simulink model "biox"  (Simulink 7.6)
settings: Solver=ode45  SolverMode=SingleTasking  StartTime=0.0  StopTime=200.0  MaxStep=0.1  RelTol=1e-9  AbsTol=1e-12
settings Model: Creator=fforbes  LastModifiedBy=fforbes  ExtModeTrigMode=oneshot  ExtModeArmWhenConnect=off
settings SolverCC: InitialStep=0.1
settings DataIOCC: LimitDataPoints=off
settings OptimizationCC: BlockReduction=off  BooleanDataType=off
settings DebuggingCC: SaveWithParameterizedLinksMsg=none  SignalResolutionControl=TryResolveAllWithWarning  SolverPrmCheckMsg=none  MultiTaskDSMMsg=warning  MultiTaskCondExecSysMsg=none  StrictBusMsg=None
settings HardwareCC: TargetUnknown=on
settings RTWCC: IncludeERTFirstTime=on

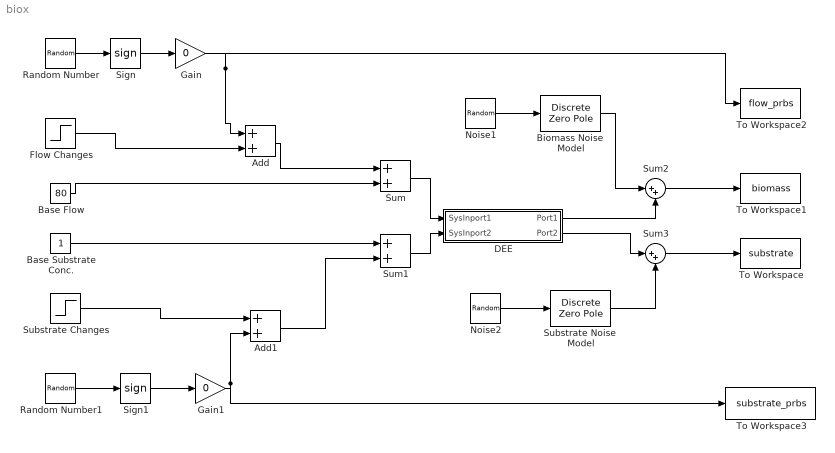
== system biox ==
  Add : Sum
  Add1 : Sum
  Base Flow : Constant  Value=80
  Base Substrate Conc. : Constant
  Biomass Noise  Model : DiscreteZeroPole  Zeros=[0.5]  Poles=[0 0.4 1]  Gain=.01
  DEE : Subsystem
      settings: OpenFcn=diffeqed
      mask Type: Differential Equation Editor (DEE)
      mask Display: disp('BIOX Unit')
  Flow Changes : Step  Time=5  After=0  SampleTime=0
  Gain : Gain  Gain=0
  Gain1 : Gain  Gain=0
  Noise1 : RandomNumber  Variance=0.00001  SampleTime=0.1
  Noise2 : RandomNumber  Variance=0.00000001  SampleTime=0.1
  Random Number : RandomNumber  SampleTime=1
  Random Number1 : RandomNumber  SampleTime=1
  Sign : Signum
  Sign1 : Signum
  Substrate Changes : Step  Time=5  After=0  SampleTime=0
  Substrate Noise  Model : DiscreteZeroPole  Zeros=[0.5]  Poles=[0.2 0.8]  Gain=1
  Sum : Sum  SaturateOnIntegerOverflow=on  InputSameDT=on  OutDataTypeStr=Inherit: Same as first input
  Sum1 : Sum  SaturateOnIntegerOverflow=on  InputSameDT=on  OutDataTypeStr=Inherit: Same as first input
  Sum2 : Sum  Inputs=|++  SaturateOnIntegerOverflow=on  InputSameDT=on  OutDataTypeStr=Inherit: Same as first input
  Sum3 : Sum  Inputs=|++  SaturateOnIntegerOverflow=on  InputSameDT=on  OutDataTypeStr=Inherit: Same as first input
  To Workspace : ToWorkspace  VariableName=substrate  SampleTime=-1  SaveFormat=Array
  To Workspace1 : ToWorkspace  VariableName=biomass  SampleTime=-1  SaveFormat=Array
  To Workspace2 : ToWorkspace  VariableName=flow_prbs  SaveFormat=Array
  To Workspace3 : ToWorkspace  VariableName=substrate_prbs  SaveFormat=Array
  wires:
  Base Substrate Conc./1 -> Sum1/1
  Sum1/1 -> DEE/2(SysInport2)
  Sum/1 -> DEE/1(SysInport1)
  Base Flow/1 -> Sum/2
  DEE/2(Port2) -> Sum3/1
  Sum3/1 -> To Workspace/1
  DEE/1(Port1) -> Sum2/2
  Sum2/1 -> To Workspace1/1
  Flow Changes/1 -> Add/2
  Random Number/1 -> Sign/1
  Add/1 -> Sum/1
  Sign/1 -> Gain/1
  Gain/1 -> Add/1, To Workspace2/1
  Random Number1/1 -> Sign1/1
  Sign1/1 -> Gain1/1
  Substrate Changes/1 -> Add1/1
  Gain1/1 -> Add1/2, To Workspace3/1
  Add1/1 -> Sum1/2
  Biomass Noise  Model/1 -> Sum2/1
  Noise1/1 -> Biomass Noise  Model/1
  Noise2/1 -> Substrate Noise  Model/1
  Substrate Noise  Model/1 -> Sum3/2

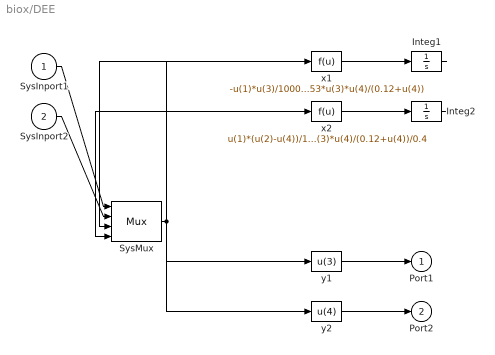
== system biox/DEE ==
  SysInport1 : Inport
  SysInport2 : Inport  Port=2
  Integ1 : Integrator  InitialCondition=0.39146666
  Integ2 : Integrator  InitialCondition=0.02133333
  SysMux : Mux
  x1 : Fcn  Expr=-u(1)*u(3)/1000+0.53*u(3)*u(4)/(0.12+u(4))
  x2 : Fcn  Expr=u(1)*(u(2)-u(4))/1000-0.53*u(3)*u(4)/(0.12+u(4))/0.4
  y1 : Fcn  Expr=u(3)
  y2 : Fcn  Expr=u(4)
  Port1 : Outport  InitialOutput=0
  Port2 : Outport  Port=2  InitialOutput=0
  wires:
  SysInport1/1 -> SysMux/1
  SysInport2/1 -> SysMux/2
  SysMux/1 -> x1/1, x2/1, y1/1, y2/1
  x1/1 -> Integ1/1
  Integ1/1 -> SysMux/3
  x2/1 -> Integ2/1
  Integ2/1 -> SysMux/4
  y1/1 -> Port1/1
  y2/1 -> Port2/1
